simulink model "SystemLoop"  (R2023a)
settings: Solver=VariableStepAuto  StartTime=0.0  StopTime=20  RelTol=1e-3
undefined symbols (not defined in the file or in its folder): A, B, C, Kp, L_o, Ts
libraries: mbedblockslib x3, stm_qeplib x1
settings Model: Creator=marco  LastModifiedBy=Marco
settings OptimizationCC: ReuseModelBlockBuffer=off

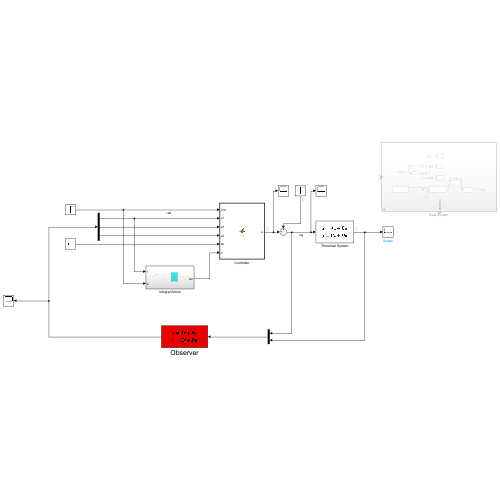
[thumbnail: Simulink's stored preview of the top-level diagram]
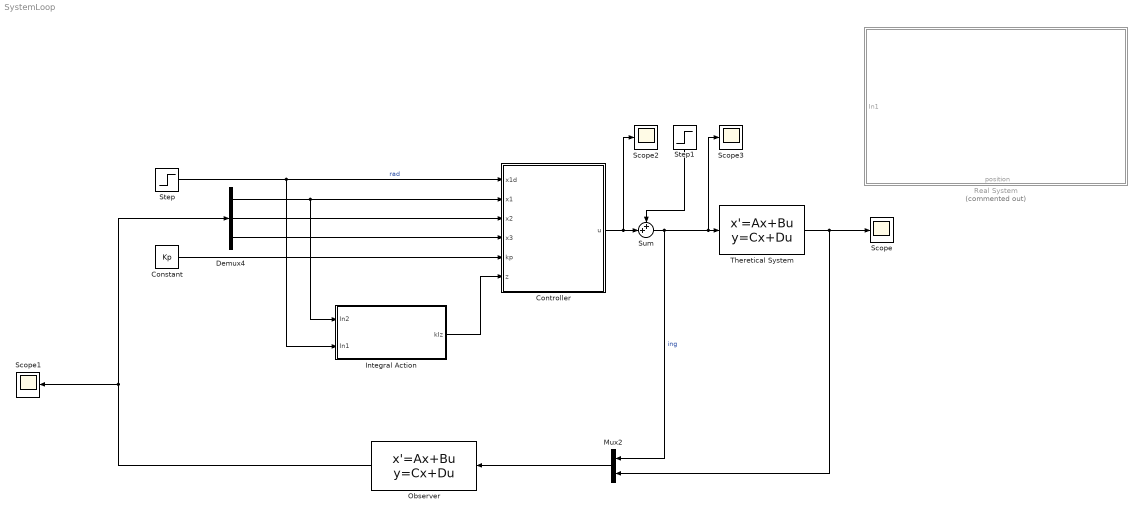
== system SystemLoop ==
  Constant : Constant  Value=Kp
  Controller : MATLAB Function  TreatAsAtomicUnit=on
  Demux4 : Demux  Outputs=3
  Integral Action : Subsystem
  Mux2 : Mux  Inputs=2
  Observer : StateSpace  A=A-L_o*C  B=[B L_o]  C=eye(3)  D=[ 0 0; 0 0; 0 0]  InitialCondition=0
  Real System : Subsystem  Commented=on
      settings: PortSchema="{\"entries\":[{\"content\":{\"sides\":[{\"content\":{\"connectorIds\":[\"In1\"]},\"type\":\"ConnectorPlacement.EquallySpacedRectSide\",\"uuid\":\"9a755849-c754-4e35-a676-7c42dc5bd414\"},{\"content\":{\"side\":\"RIGHT\"},\"type\":\"ConnectorPlacement.EquallySpacedRectSide\",\"uuid\":\"44a7a0a1-1ee9-4c14-b80d-a747da089048\"},{\"content\":{\"side\":\"TOP\"},\"type\":\"ConnectorPlacement.EquallySpacedRectSide\",\"uuid\":\"b200f8ea-5786-4ccf-a609-f78dac3fdfe3\"},{\"content\":{\"connectorIds\":[\"Out1\"],\"side\":\"BOTTOM\"},\"type\":\"ConnectorPlacement.EquallySpacedRectSide\",\"uuid\":\"0b26f2bc-f6b7-41a0-8206-00c2b8e147b9\"}]},\"type\":\"ConnectorPlacement.EquallySpacedConnector\",\"uuid\":\"4c1c8d1a-48cf-4ac5-ad5e-29d8d7fb8083\"}],\"packageUris\":[\"http://schema.mathworks.com/mf0/Connector/R2020b\"],\"version\":\"1.0\"}"
  Scope{,1..3} (4 alike) : Scope
  Step : Step  Time=0  After=deg2rad(180)  SampleTime=0
  Step1 : Step  After=0.5  SampleTime=0
  Sum : Sum  Inputs=++|
  Theretical System : StateSpace  A=A  B=B  C=C  D=0  InitialCondition=0
  wires:
  Step/1 -> Integral Action/2(In1), Controller/1(x1d)  "rad"
  Constant/1 -> Controller/5(kp)
  Theretical System/1 -> Mux2/2, Scope/1
  Mux2/1 -> Observer/1
  Observer/1 -> Demux4/1, Scope1/1
  Step1/1 -> Sum/1
  Controller/1(u) -> Scope2/1, Sum/2
  Demux4/1 -> Integral Action/1(In2), Controller/2(x1)
  Demux4/2 -> Controller/3(x2)
  Demux4/3 -> Controller/4(x3)
  Sum/1 -> Scope3/1, Theretical System/1, Mux2/1  "ing"
  Integral Action/1(kIz) -> Controller/6(z)

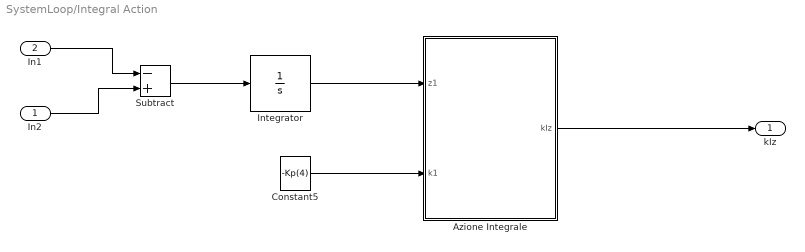
== system SystemLoop/Integral Action ==
  In2 : Inport
  In1 : Inport  Port=2
  Azione Integrale : MATLAB Function  TreatAsAtomicUnit=on
  Constant5 : Constant  Value=-Kp(4)
  Integrator : Integrator
  Subtract : Sum  Inputs=-+
  kIz : Outport
  wires:
  Integrator/1 -> Azione Integrale/1(z1)
  Constant5/1 -> Azione Integrale/2(k1)
  Subtract/1 -> Integrator/1
  In1/1 -> Subtract/1
  Azione Integrale/1(kIz) -> kIz/1
  In2/1 -> Subtract/2

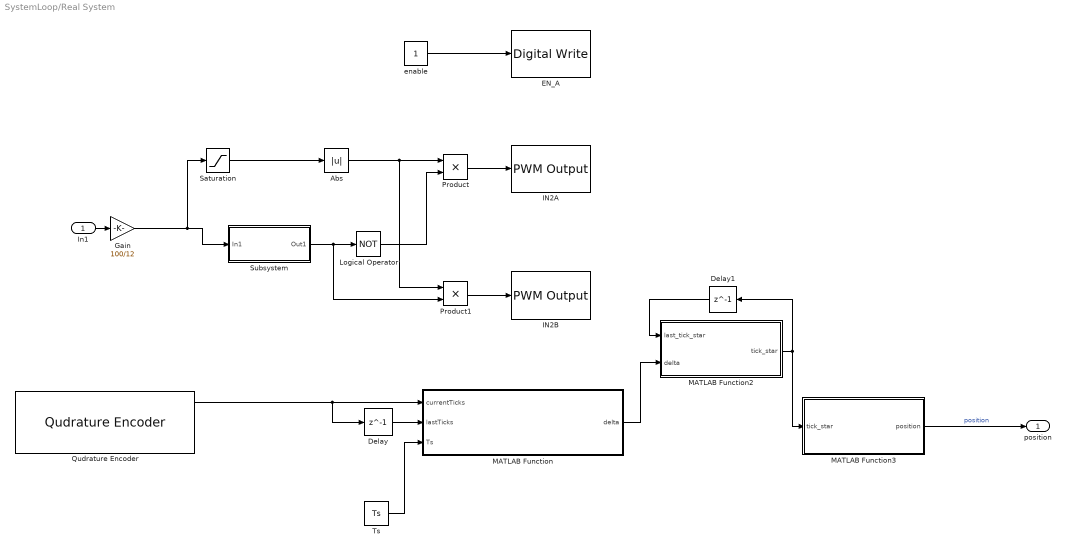
== system SystemLoop/Real System ==
  In1 : Inport
  Abs : Abs  SaturateOnIntegerOverflow=off
  Delay : Delay  DelayLength=1  InitialCondition=0
  Delay1 : Delay  DelayLength=1  InitialCondition=0
  EN_A : mbedblockslib/Digital Write  Pin=2  Direction=output
      settings: LibrarySourceBlock=stmnucleorootlib/Common/Digital Write
  Gain : Gain  Gain=100/12
  IN2A : mbedblockslib/PWM Output  Pin=4  EnableInputFrequency=off  InitialFrequency=PWMFreq  InitialDutyCycle=50  NotificationType=None
      settings: LibrarySourceBlock=stmnucleorootlib/Common/PWM Output
  IN2B : mbedblockslib/PWM Output  Pin=5  EnableInputFrequency=off  InitialFrequency=PWMFreq  InitialDutyCycle=50  NotificationType=None
      settings: LibrarySourceBlock=stmnucleorootlib/Common/PWM Output
  Logical Operator : Logic  Operator=NOT  AllPortsSameDT=off  OutDataTypeStr=boolean
  MATLAB Function : MATLAB Function  TreatAsAtomicUnit=on
  MATLAB Function2 : MATLAB Function  TreatAsAtomicUnit=on
  MATLAB Function3 : MATLAB Function  TreatAsAtomicUnit=on
  Product : Product
  Product1 : Product
  Qudrature Encoder : stm_qeplib/Qudrature Encoder  SampleTime=Ts
  Saturation : Saturate  UpperLimit=100  LowerLimit=-100
  Subsystem : Subsystem
  Ts : Constant  Value=Ts
  enable : Constant
  position : Outport
  wires:
  enable/1 -> EN_A/1
  Subsystem/1(Out1) -> Product1/2, Logical Operator/1
  Saturation/1 -> Abs/1
  Product1/1 -> IN2B/1
  Product/1 -> IN2A/1
  Logical Operator/1 -> Product/2
  Abs/1 -> Product1/1, Product/1
  Gain/1 -> Saturation/1, Subsystem/1(In1)
  MATLAB Function2/1(tick_star) -> MATLAB Function3/1(tick_star), Delay1/1
  Qudrature Encoder/1 -> Delay/1, MATLAB Function/1(currentTicks)
  MATLAB Function/1(delta) -> MATLAB Function2/2(delta)
  Delay1/1 -> MATLAB Function2/1(last_tick_star)
  Ts/1 -> MATLAB Function/3(Ts)
  Delay/1 -> MATLAB Function/2(lastTicks)
  In1/1 -> Gain/1
  MATLAB Function3/1(position) -> position/1  "position"

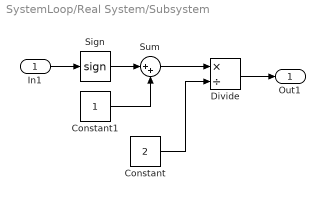
== system SystemLoop/Real System/Subsystem ==
  In1 : Inport
  Constant : Constant  Value=2
  Constant1 : Constant
  Divide : Product  Inputs=*/
  Sign : Signum
  Sum : Sum  Inputs=|++
  Out1 : Outport
  wires:
  In1/1 -> Sign/1
  Sign/1 -> Sum/1
  Constant1/1 -> Sum/2
  Sum/1 -> Divide/1
  Constant/1 -> Divide/2
  Divide/1 -> Out1/1

== matlab function SystemLoop/Real System/MATLAB Function ==
  data: currentTicks input; delta output; lastTicks input; Ts input
function delta = getTicksDelta(currentTicks, lastTicks, Ts)

currentTicks = double(currentTicks);
lastTicks = double(lastTicks);

if abs(currentTicks - lastTicks) <= ceil(8400*Ts)
    delta = currentTicks-lastTicks;
else
    if lastTicks > currentTicks
        delta = currentTicks + 2^16-1-lastTicks;
    else
        delta = currentTicks - 2^16+1-lastTicks;

end

end

== matlab function SystemLoop/Controller ==
  data: x1d input; x1 input; u output; x2 input; x3 input; kp input; z input
function u = fcn(x1d, x1, x2, x3, kp, z)

c = -kp(1)*(x1-x1d) - kp(2)*x2 - kp(3)*x3 + z;

if c>12
    c = 12
elseif c<-12
    c = -12
end

u = c

== matlab function SystemLoop/Integral Action/Azione Integrale ==
  data: z1 input; kIz output; k1 input
function kIz = fcn(z1, k1)

kIz = z1*k1

== matlab function SystemLoop/Real System/MATLAB Function2 ==
  data: last_tick_star input; delta input; tick_star output
function tick_star = modCounter(last_tick_star, delta)

    % 89796 numero di tick per effettuare 25 giri completo
    tick_star = mod(last_tick_star + delta, 89796)

end

== matlab function SystemLoop/Real System/MATLAB Function3 ==
  data: tick_star input; position output
function position = getPosition(tick_star)

    tick_star = double(tick_star);

    completeTheta = 2*pi*tick_star/(3591.84);

    position = sign(completeTheta) * mod(abs(completeTheta), 2*pi);

end
